simulink model "DahlinovPID"  (R2016a)
settings: Solver=VariableStepAuto  SolverMode=SingleTasking  StartTime=0.0  StopTime=50  RelTol=1e-3
values from neighbouring files (symbols this model uses):
  K = 0.0741    [Parameters.m]
  Kp = -253.9209    [Parameters.m]
  M = 1.8018    [Parameters.m]
settings Model: Creator=User  LastModifiedBy=M-Pc
settings DebuggingCC: SFUnexpectedBacktrackingDiag=error  SFNoUnconditionalDefaultTransitionDiag=error
settings GRTTargetCC: TargetLangStandard=C99 (ISO)  GeneratePreprocessorConditionals=Use local settings
settings ConfigComp: CovMetricSettings=dwe  CovHtmlReporting=off  CovSaveCumulativeToWorkspaceVar=off  CovSaveSingleToWorkspaceVar=off  CovExternalEMLEnable=on

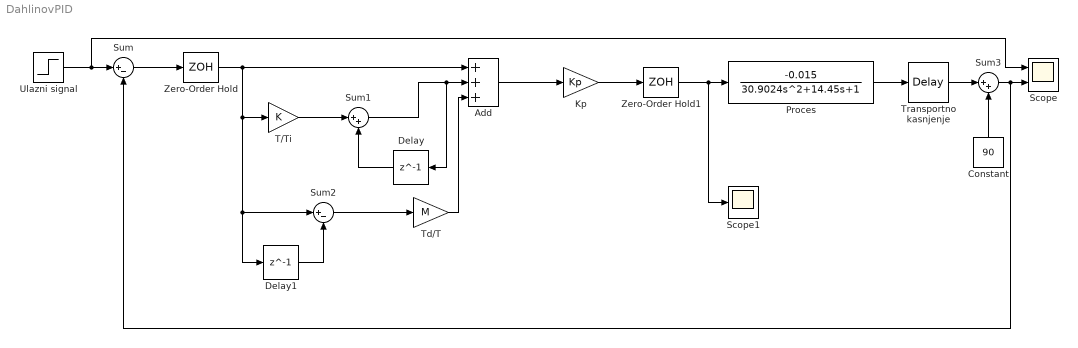
== system DahlinovPID ==
  Add : Sum  Inputs=+++
  Constant : Constant  Value=90
  Delay : Delay  DelayLength=1
  Delay1 : Delay  DelayLength=1
  Kp : Gain  Gain=Kp
  Proces : TransferFcn  Numerator=[-0.015]  Denominator=[30.9024 14.45 1]
  Scope : Scope  NumInputPorts=2
  Scope1 : Scope
  Sum : Sum  Inputs=|+-
  Sum1 : Sum  Inputs=|++
  Sum2 : Sum  Inputs=|+-
  Sum3 : Sum  Inputs=|++
  T/Ti : Gain  Gain=K
  Td/T : Gain  Gain=M
  Transportno kasnjenje : TransportDelay
  Ulazni signal : Step  Time=5  Before=90  After=80  SampleTime=0
  Zero-Order Hold : ZeroOrderHold
  Zero-Order Hold1 : ZeroOrderHold
  wires:
  Ulazni signal/1 -> Scope/1, Sum/1
  Sum/1 -> Zero-Order Hold/1
  Zero-Order Hold/1 -> Sum2/1, Delay1/1, T/Ti/1, Add/1
  T/Ti/1 -> Sum1/1
  Sum1/1 -> Delay/1, Add/2
  Delay/1 -> Sum1/2
  Delay1/1 -> Sum2/2
  Sum2/1 -> Td/T/1
  Td/T/1 -> Add/3
  Add/1 -> Kp/1
  Kp/1 -> Zero-Order Hold1/1
  Zero-Order Hold1/1 -> Scope1/1, Proces/1
  Proces/1 -> Transportno kasnjenje/1
  Transportno kasnjenje/1 -> Sum3/1
  Constant/1 -> Sum3/2
  Sum3/1 -> Sum/2, Scope/2
